simulink model "model_1_type"  (R2022b)
settings: Solver=VariableStepAuto  StartTime=0.0  StopTime=2000  MaxStep=1e-3  RelTol=1e-3
undefined symbols (not defined in the file or in its folder): a0, a1, b0, gamma, k0, k_M_1, k_M_2
settings Model: Creator=deniskirbaba  LastModifiedBy=R1303-We2-1-Stud
settings OptimizationCC: ReuseModelBlockBuffer=on

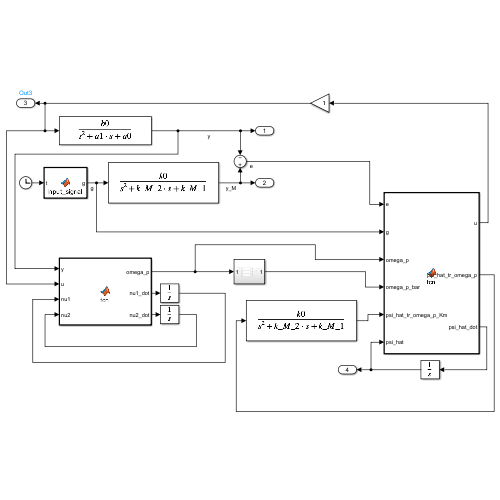
[thumbnail: Simulink's stored preview of the top-level diagram]
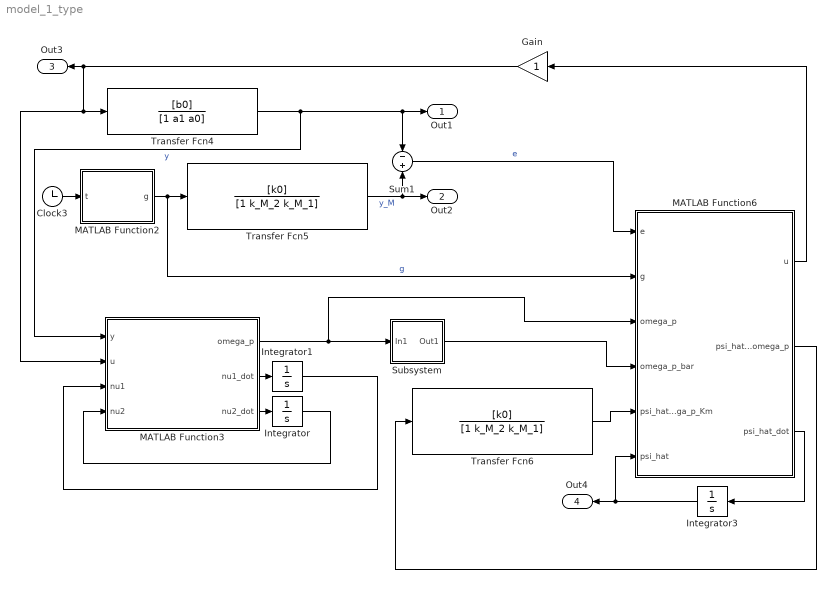
== system model_1_type ==
  Clock3 : Clock
  Gain : Gain
  Integrator : Integrator
  Integrator1 : Integrator
  Integrator3 : Integrator  InitialCondition=[0;0;0]
  MATLAB Function2 : MATLAB Function  TreatAsAtomicUnit=on
  MATLAB Function3 : MATLAB Function  TreatAsAtomicUnit=on
  MATLAB Function6 : MATLAB Function  TreatAsAtomicUnit=on
  Subsystem : Subsystem
  Sum1 : Sum  Inputs=-+
  Transfer Fcn4 : TransferFcn  Numerator=[b0]  Denominator=[1 a1 a0]
  Transfer Fcn5 : TransferFcn  Numerator=[k0]  Denominator=[1 k_M_2 k_M_1]
  Transfer Fcn6 : TransferFcn  Numerator=[k0]  Denominator=[1 k_M_2 k_M_1]
  Out1 : Outport
  Out2 : Outport  Port=2
  Out3 : Outport  Port=3
  Out4 : Outport  Port=4
  wires:
  Clock3/1 -> MATLAB Function2/1(t)
  MATLAB Function2/1(g) -> MATLAB Function6/2(g), Transfer Fcn5/1  "g"
  Transfer Fcn5/1 -> Out2/1, Sum1/2  "y_M"
  Transfer Fcn4/1 -> MATLAB Function3/1(y), Out1/1, Sum1/1  "y"
  Sum1/1 -> MATLAB Function6/1(e)  "e"
  MATLAB Function3/3(nu2_dot) -> Integrator/1
  MATLAB Function3/2(nu1_dot) -> Integrator1/1
  Integrator/1 -> MATLAB Function3/4(nu2)
  Integrator1/1 -> MATLAB Function3/3(nu1)
  MATLAB Function3/1(omega_p) -> MATLAB Function6/3(omega_p), Subsystem/1(In1)
  Subsystem/1(Out1) -> MATLAB Function6/4(omega_p_bar)
  MATLAB Function6/3(psi_hat_dot) -> Integrator3/1
  Integrator3/1 -> MATLAB Function6/6(psi_hat), Out4/1
  MATLAB Function6/2(psi_hat_tr_omega_p) -> Transfer Fcn6/1
  Transfer Fcn6/1 -> MATLAB Function6/5(psi_hat_tr_omega_p_Km)
  MATLAB Function6/1(u) -> Gain/1
  Gain/1 -> Out3/1, MATLAB Function3/2(u), Transfer Fcn4/1

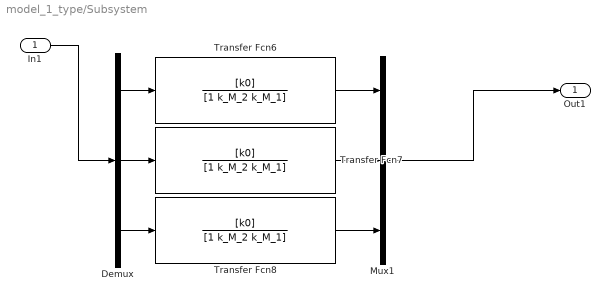
== system model_1_type/Subsystem ==
  In1 : Inport
  Demux : Demux  Outputs=3
  Mux1 : Mux  Inputs=3
  Transfer Fcn6 : TransferFcn  Numerator=[k0]  Denominator=[1 k_M_2 k_M_1]
  Transfer Fcn7 : TransferFcn  Numerator=[k0]  Denominator=[1 k_M_2 k_M_1]
  Transfer Fcn8 : TransferFcn  Numerator=[k0]  Denominator=[1 k_M_2 k_M_1]
  Out1 : Outport
  wires:
  Transfer Fcn6/1 -> Mux1/1
  Demux/1 -> Transfer Fcn6/1
  Demux/3 -> Transfer Fcn8/1
  Demux/2 -> Transfer Fcn7/1
  Transfer Fcn7/1 -> Mux1/2
  In1/1 -> Demux/1
  Mux1/1 -> Out1/1
  Transfer Fcn8/1 -> Mux1/3

== matlab function model_1_type/MATLAB Function2 ==
  data: t input; g output
function g = input_signal(t)
    g = 7*sign(cos(0.9*t));
end

== matlab function model_1_type/MATLAB Function3 ==
  data: y input; u input; nu1 input; nu2 input; omega_p output; nu1_dot output; nu2_dot output; k0 parameter
function [omega_p, nu1_dot, nu2_dot] = fcn(y, u, nu1, nu2, k0)
    lambda =-k0;
    
    nu1_dot = lambda*nu1 + u;
    nu2_dot = lambda*nu2 + y;

    omega = [nu1',nu2',y]';
    omega_p = -omega;
end

== matlab function model_1_type/MATLAB Function6 ==
  data: e input; g input; omega_p input; omega_p_bar input; psi_hat_tr_omega_p_Km input; psi_hat input; u output; psi_hat_tr_omega_p output; psi_hat_dot output; k0 parameter; gamma parameter; b0 parameter
function [u, psi_hat_tr_omega_p, psi_hat_dot] = fcn(e, g, omega_p, omega_p_bar, psi_hat_tr_omega_p_Km, psi_hat, k0, gamma, b0)
    psi_hat_tr_omega_p = psi_hat'*omega_p;
    e_hat = e-psi_hat'*omega_p_bar+psi_hat_tr_omega_p_Km;
    psi_hat_dot = gamma*omega_p_bar/(1+omega_p_bar'*omega_p_bar)*e_hat;
    u = (psi_hat'*omega_p+k0*g)/b0;
end
